simulink subsystem "AntiPark"  (R2023b)
settings: Solver=VariableStepAuto  StartTime=0.0  StopTime=10.0  RelTol=1e-3
settings Model: Creator=rainy  LastModifiedBy=rainy

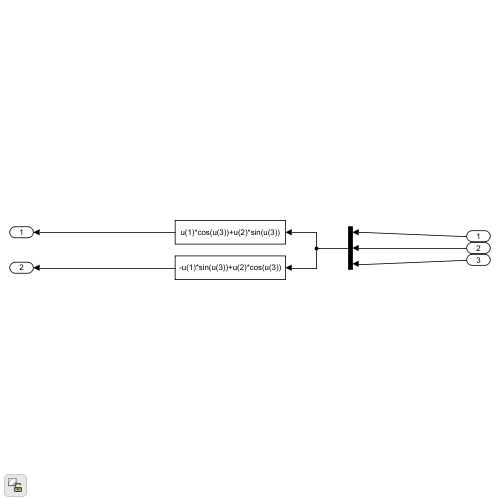
[thumbnail: Simulink's stored preview of the top-level diagram]
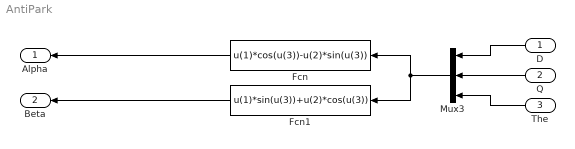
== system AntiPark ==
  D : Inport
  Q : Inport  Port=2
  The : Inport  Port=3
  Fcn : Fcn  Expr=u(1)*cos(u(3))-u(2)*sin(u(3))
  Fcn1 : Fcn  Expr=u(1)*sin(u(3))+u(2)*cos(u(3))
  Mux3 : Mux  Inputs=3
  Alpha : Outport
  Beta : Outport  Port=2
  wires:
  Mux3/1 -> Fcn/1, Fcn1/1
  Fcn/1 -> Alpha/1
  The/1 -> Mux3/3
  D/1 -> Mux3/1
  Q/1 -> Mux3/2
  Fcn1/1 -> Beta/1
